simulink model "practica2_3x3sonmem"  (Simulink 7.3)
settings: Solver=ode45  StartTime=0.0  StopTime=10.0  RelTol=1e-3
undefined symbols (not defined in the file or in its folder): p
libraries: simeventsrouting1 x15, simeventssink1 x12, simeventsgenerators1 x6, simeventsqueue1 x6, simeventsattributes2 x6, simeventstiming1 x6, simeventsgates1 x3, simeventsserver1 x3
settings Model: Creator=usuario  LastModifiedBy=usuario
settings SimEventsCC: propDiagAttribOutput=1  propDiagFcnCallOutput=1  propDiagStatOutput=0

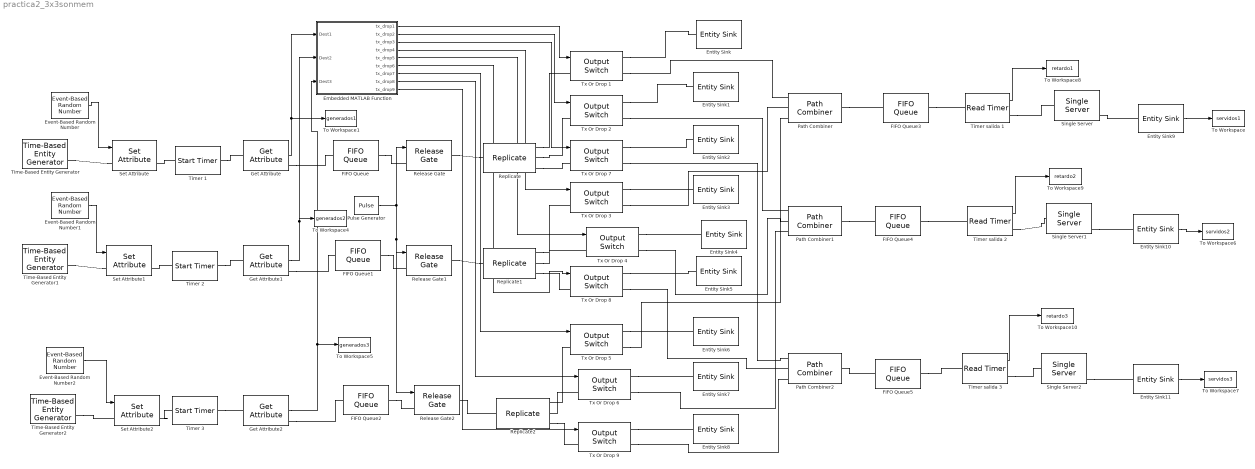
== system practica2_3x3sonmem ==
  Embedded MATLAB Function : Stateflow chart
  Entity Sink{,1..8} (9 alike) : simeventssink1/Entity Sink  Priority=1  SystemSampleTime=-1  AvailableForArrivals=on  StatNumberArrived=Off
  Entity Sink10 : simeventssink1/Entity Sink  Priority=1  SystemSampleTime=-1  AvailableForArrivals=on  StatNumberArrived=On
  Entity Sink11 : simeventssink1/Entity Sink  Priority=1  SystemSampleTime=-1  AvailableForArrivals=on  StatNumberArrived=On
  Entity Sink9 : simeventssink1/Entity Sink  Priority=1  SystemSampleTime=-1  AvailableForArrivals=on  StatNumberArrived=On
  Event-Based Random Number : simeventsgenerators1/Signal Generators/Event-Based Random Number  SystemSampleTime=-1  distribution=Arbitrary discrete  meanExp=1  minUnif=1  maxUnif=1  pOneBern=0.25  pSuccessBino=0.5  numTrialBino=1  meanNorm=0  stdNorm=1  minTri=1  maxTri=3  modeTri=2  thresholdLogn=0  scaleLogn=1  shapeLogn=1  pSuccessGeo=0.5  meanPoiss=1  thresholdLogl=0  scaleLogl=1  thresholdGam=0  scaleGam=1  shapeGam=1  minBeta=0  maxBeta=1  shape1Beta=1  shape2Beta=1  minUnid=0  maxUnid=1  numValueUnid=2  thresholdWbl=0  scaleWbl=1  shapeWbl=1  valueVecCont=[0 1]  cdfVecCont=[0 1]  valueVecDisc=[0 1 2 3]  probVecDisc=[1-p p/3 p/3 p/3]  seed=12345  IsProcessed=on  isConnected=1
  Event-Based Random Number1 : simeventsgenerators1/Signal Generators/Event-Based Random Number  SystemSampleTime=-1  distribution=Arbitrary discrete  meanExp=1  minUnif=1  maxUnif=1  pOneBern=0.25  pSuccessBino=0.5  numTrialBino=1  meanNorm=0  stdNorm=1  minTri=1  maxTri=3  modeTri=2  thresholdLogn=0  scaleLogn=1  shapeLogn=1  pSuccessGeo=0.5  meanPoiss=1  thresholdLogl=0  scaleLogl=1  thresholdGam=0  scaleGam=1  shapeGam=1  minBeta=0  maxBeta=1  shape1Beta=1  shape2Beta=1  minUnid=0  maxUnid=1  numValueUnid=2  thresholdWbl=0  scaleWbl=1  shapeWbl=1  valueVecCont=[0 1]  cdfVecCont=[0 1]  valueVecDisc=[0 1 2 3]  probVecDisc=[1-p p/3 p/3 p/3]  seed=76543  IsProcessed=on  isConnected=1
  Event-Based Random Number2 : simeventsgenerators1/Signal Generators/Event-Based Random Number  SystemSampleTime=-1  distribution=Arbitrary discrete  meanExp=1  minUnif=1  maxUnif=1  pOneBern=0.25  pSuccessBino=0.5  numTrialBino=1  meanNorm=0  stdNorm=1  minTri=1  maxTri=3  modeTri=2  thresholdLogn=0  scaleLogn=1  shapeLogn=1  pSuccessGeo=0.5  meanPoiss=1  thresholdLogl=0  scaleLogl=1  thresholdGam=0  scaleGam=1  shapeGam=1  minBeta=0  maxBeta=1  shape1Beta=1  shape2Beta=1  minUnid=0  maxUnid=1  numValueUnid=2  thresholdWbl=0  scaleWbl=1  shapeWbl=1  valueVecCont=[0 1]  cdfVecCont=[0 1]  valueVecDisc=[0 1 2 3]  probVecDisc=[1-p p/3 p/3 p/3]  seed=89652  IsProcessed=on  isConnected=1
  FIFO Queue : simeventsqueue1/FIFO Queue  Priority=1  SystemSampleTime=-1  Capacity=1  EnableTOPort=off  StatNumberDeparted=Off  StatNumberInBlock=Off  StatPendingEntity=Off  StatAverageWait=Off  StatAverageQueueLength=Off  StatNumberTimedout=Off
  FIFO Queue1 : simeventsqueue1/FIFO Queue  Priority=1  SystemSampleTime=-1  Capacity=1  EnableTOPort=off  StatNumberDeparted=Off  StatNumberInBlock=Off  StatPendingEntity=Off  StatAverageWait=Off  StatAverageQueueLength=Off  StatNumberTimedout=Off
  FIFO Queue2 : simeventsqueue1/FIFO Queue  Priority=1  SystemSampleTime=-1  Capacity=1  EnableTOPort=off  StatNumberDeparted=Off  StatNumberInBlock=Off  StatPendingEntity=Off  StatAverageWait=Off  StatAverageQueueLength=Off  StatNumberTimedout=Off
  FIFO Queue3 : simeventsqueue1/FIFO Queue  Priority=1  SystemSampleTime=-1  Capacity=100  EnableTOPort=off  StatNumberDeparted=Off  StatNumberInBlock=Off  StatPendingEntity=Off  StatAverageWait=Off  StatAverageQueueLength=Off  StatNumberTimedout=Off
  FIFO Queue4 : simeventsqueue1/FIFO Queue  Priority=1  SystemSampleTime=-1  Capacity=100  EnableTOPort=off  StatNumberDeparted=Off  StatNumberInBlock=Off  StatPendingEntity=Off  StatAverageWait=Off  StatAverageQueueLength=Off  StatNumberTimedout=Off
  FIFO Queue5 : simeventsqueue1/FIFO Queue  Priority=1  SystemSampleTime=-1  Capacity=100  EnableTOPort=off  StatNumberDeparted=Off  StatNumberInBlock=Off  StatPendingEntity=Off  StatAverageWait=Off  StatAverageQueueLength=Off  StatNumberTimedout=Off
  Get Attribute : simeventsattributes2/Get Attribute  Priority=1  DialogController=des_ddg_create  DialogControllerArgs=DataTag19  SystemSampleTime=-1  AttributeName=Attribute1  AttributeMissing=Error  AttributeDefaultValue=1  AttributeSendTiming=After entity departure  AttributeTreatAsVector=1  StatNumberDeparted=On  EvaluatedDefaultAttributeValue={[]}
  Get Attribute1 : simeventsattributes2/Get Attribute  Priority=1  DialogController=des_ddg_create  DialogControllerArgs=DataTag21  SystemSampleTime=-1  AttributeName=Attribute1  AttributeMissing=Error  AttributeDefaultValue=1  AttributeSendTiming=After entity departure  AttributeTreatAsVector=1  StatNumberDeparted=On  EvaluatedDefaultAttributeValue={[]}
  Get Attribute2 : simeventsattributes2/Get Attribute  Priority=1  DialogController=des_ddg_create  DialogControllerArgs=DataTag23  SystemSampleTime=-1  AttributeName=Attribute1  AttributeMissing=Error  AttributeDefaultValue=1  AttributeSendTiming=After entity departure  AttributeTreatAsVector=1  StatNumberDeparted=On  EvaluatedDefaultAttributeValue={[]}
  Path Combiner : simeventsrouting1/Path Combiner  Priority=1  SystemSampleTime=-1  NumberInputPorts=3  InputPortPrecedence=IN1 port  InitialSeed=45675  SpecifyEventPriority=off  PriorityPathCombinerPortPrecedenceSelection=4100  StatNumberDeparted=Off  StatLastArrivalPort=Off  EvaluatedNumPorts=3
  Path Combiner1 : simeventsrouting1/Path Combiner  Priority=1  SystemSampleTime=-1  NumberInputPorts=3  InputPortPrecedence=IN1 port  InitialSeed=45675  SpecifyEventPriority=off  PriorityPathCombinerPortPrecedenceSelection=4100  StatNumberDeparted=Off  StatLastArrivalPort=Off  EvaluatedNumPorts=3
  Path Combiner2 : simeventsrouting1/Path Combiner  Priority=1  SystemSampleTime=-1  NumberInputPorts=3  InputPortPrecedence=IN1 port  InitialSeed=45675  SpecifyEventPriority=off  PriorityPathCombinerPortPrecedenceSelection=4100  StatNumberDeparted=Off  StatLastArrivalPort=Off  EvaluatedNumPorts=3
  Pulse Generator : DiscretePulseGenerator  Amplitude=1  Period=10  PulseWidth=5  PhaseDelay=3  SampleTime=0.1
  Release Gate : simeventsgates1/Release Gate  Priority=1  SystemSampleTime=-1  OpenGateUpon=Change in signal from port vc  SignalEdgeOption=Rising  SpecifyEventPriority=off  PriorityGateRelease=2200  StatNumberDeparted=Off
  Release Gate1 : simeventsgates1/Release Gate  Priority=1  SystemSampleTime=-1  OpenGateUpon=Change in signal from port vc  SignalEdgeOption=Rising  SpecifyEventPriority=off  PriorityGateRelease=2200  StatNumberDeparted=Off
  Release Gate2 : simeventsgates1/Release Gate  Priority=1  SystemSampleTime=-1  OpenGateUpon=Change in signal from port vc  SignalEdgeOption=Rising  SpecifyEventPriority=off  PriorityGateRelease=2200  StatNumberDeparted=Off
  Replicate : simeventsrouting1/Replicate  Priority=1  SystemSampleTime=-1  NumberOutputPorts=3  ReplicateEntityWhen=All entity output ports are not blocked  OutputPortPrecedence=OUT1 port  InitialSeed=56789  ActionUponBlocking=Discard entity  StatNumberArrived=Off  StatNumberDeparted=Off  EvaluatedNumPorts=3
  Replicate1 : simeventsrouting1/Replicate  Priority=1  SystemSampleTime=-1  NumberOutputPorts=3  ReplicateEntityWhen=All entity output ports are not blocked  OutputPortPrecedence=OUT1 port  InitialSeed=56789  ActionUponBlocking=Discard entity  StatNumberArrived=Off  StatNumberDeparted=Off  EvaluatedNumPorts=3
  Replicate2 : simeventsrouting1/Replicate  Priority=1  SystemSampleTime=-1  NumberOutputPorts=3  ReplicateEntityWhen=All entity output ports are not blocked  OutputPortPrecedence=OUT1 port  InitialSeed=56789  ActionUponBlocking=Discard entity  StatNumberArrived=Off  StatNumberDeparted=Off  EvaluatedNumPorts=3
  Set Attribute : simeventsattributes2/Set Attribute  Priority=1  DialogController=des_ddg_create  DialogControllerArgs=DataTag34  SystemSampleTime=-1  AttributeFrom=Signal port  AttributeName=Attribute1  AttributeTreatAsVector=1  AttributeValue=1  AttributeCreate=on  StatNumberDeparted=On  EvaluatedAttributeValue={[]}
  Set Attribute1 : simeventsattributes2/Set Attribute  Priority=1  DialogController=des_ddg_create  DialogControllerArgs=DataTag36  SystemSampleTime=-1  AttributeFrom=Signal port  AttributeName=Attribute1  AttributeTreatAsVector=1  AttributeValue=1  AttributeCreate=on  StatNumberDeparted=On  EvaluatedAttributeValue={[]}
  Set Attribute2 : simeventsattributes2/Set Attribute  Priority=1  DialogController=des_ddg_create  DialogControllerArgs=DataTag38  SystemSampleTime=-1  AttributeFrom=Signal port  AttributeName=Attribute1  AttributeTreatAsVector=1  AttributeValue=1  AttributeCreate=on  StatNumberDeparted=On  EvaluatedAttributeValue={[]}
  Single Server : simeventsserver1/Single Server  Priority=1  SystemSampleTime=-1  ServiceTimeFrom=Dialog  ServiceTime=0.99999  AttributeName=ServiceTime  PriorityServiceCompletion=500  PermitPreemption=off  SortingAttributeName=PriorityAttributeName  SortingDirection=Ascending  WriteToAttribute=off  ResidualAttributeName=ResidualServiceTime  CreateAttribute=on  EnableTOPort=off  StatNumberDeparted=On  StatNumberInBlock=Off  StatNumberPreempted=Off  StatPendingEntity=Off  StatAverageWait=Off  StatUtilization=On  StatNumberTimedout=Off
  Single Server1 : simeventsserver1/Single Server  Priority=1  SystemSampleTime=-1  ServiceTimeFrom=Dialog  ServiceTime=0.99999  AttributeName=ServiceTime  PriorityServiceCompletion=500  PermitPreemption=off  SortingAttributeName=PriorityAttributeName  SortingDirection=Ascending  WriteToAttribute=off  ResidualAttributeName=ResidualServiceTime  CreateAttribute=on  EnableTOPort=off  StatNumberDeparted=On  StatNumberInBlock=Off  StatNumberPreempted=Off  StatPendingEntity=Off  StatAverageWait=Off  StatUtilization=On  StatNumberTimedout=Off
  Single Server2 : simeventsserver1/Single Server  Priority=1  SystemSampleTime=-1  ServiceTimeFrom=Dialog  ServiceTime=0.99999  AttributeName=ServiceTime  PriorityServiceCompletion=500  PermitPreemption=off  SortingAttributeName=PriorityAttributeName  SortingDirection=Ascending  WriteToAttribute=off  ResidualAttributeName=ResidualServiceTime  CreateAttribute=on  EnableTOPort=off  StatNumberDeparted=On  StatNumberInBlock=Off  StatNumberPreempted=Off  StatPendingEntity=Off  StatAverageWait=Off  StatUtilization=On  StatNumberTimedout=Off
  Time-Based Entity Generator : simeventsgenerators1/Entity Generators/Time-Based Entity Generator  Priority=1  DialogController=des_ddg_create  DialogControllerArgs=DataTag43  SystemSampleTime=-1  GenerateEntitiesUpon=Intergeneration time from dialog  Distribution=Constant  Minimum=0  Maximum=1  Mean=1  InitialSeed=12345  Period=1  PriorityEntityGeneration=300  GenerateEntityAtSimulationStart=on  ResponseWhenBlocked=Pause generation  ResponseWhenUnblocked=Immediate restart  EntityType=Blank  StatNumberDeparted=On  StatPendingEntity=Off  StatAverageIntergenerationTime=Off
  Time-Based Entity Generator1 : simeventsgenerators1/Entity Generators/Time-Based Entity Generator  Priority=1  DialogController=des_ddg_create  DialogControllerArgs=DataTag45  SystemSampleTime=-1  GenerateEntitiesUpon=Intergeneration time from dialog  Distribution=Constant  Minimum=0  Maximum=1  Mean=1  InitialSeed=12345  Period=1  PriorityEntityGeneration=300  GenerateEntityAtSimulationStart=on  ResponseWhenBlocked=Pause generation  ResponseWhenUnblocked=Immediate restart  EntityType=Blank  StatNumberDeparted=On  StatPendingEntity=Off  StatAverageIntergenerationTime=Off
  Time-Based Entity Generator2 : simeventsgenerators1/Entity Generators/Time-Based Entity Generator  Priority=1  DialogController=des_ddg_create  DialogControllerArgs=DataTag47  SystemSampleTime=-1  GenerateEntitiesUpon=Intergeneration time from dialog  Distribution=Constant  Minimum=0  Maximum=1  Mean=1  InitialSeed=12345  Period=1  PriorityEntityGeneration=300  GenerateEntityAtSimulationStart=on  ResponseWhenBlocked=Pause generation  ResponseWhenUnblocked=Immediate restart  EntityType=Blank  StatNumberDeparted=On  StatPendingEntity=Off  StatAverageIntergenerationTime=Off
  Timer 1 : simeventstiming1/Start Timer  Priority=0  SystemSampleTime=-1  TimerTag=T1  TimerStartedOption=Warn and continue  StatNumberDeparted=Off
  Timer 2 : simeventstiming1/Start Timer  Priority=0  SystemSampleTime=-1  TimerTag=T1  TimerStartedOption=Warn and continue  StatNumberDeparted=Off
  Timer 3 : simeventstiming1/Start Timer  Priority=0  SystemSampleTime=-1  TimerTag=T1  TimerStartedOption=Warn and continue  StatNumberDeparted=Off
  Timer salida 1 : simeventstiming1/Read Timer  Priority=0  SystemSampleTime=-1  TimerTag=T1  TimerModeOption=Error  TimerStop=off  StatNumberDeparted=Off  StatTimerNumberDeparted=Off  StatTimeElapsed=On  StatAverageTimeElapsed=Off
  Timer salida 2 : simeventstiming1/Read Timer  Priority=0  SystemSampleTime=-1  TimerTag=T1  TimerModeOption=Error  TimerStop=off  StatNumberDeparted=Off  StatTimerNumberDeparted=Off  StatTimeElapsed=On  StatAverageTimeElapsed=Off
  Timer salida 3 : simeventstiming1/Read Timer  Priority=0  SystemSampleTime=-1  TimerTag=T1  TimerModeOption=Error  TimerStop=off  StatNumberDeparted=Off  StatTimerNumberDeparted=Off  StatTimeElapsed=On  StatAverageTimeElapsed=Off
  To Workspace : ToWorkspace  VariableName=servidos1  SampleTime=-1  SaveFormat=Array
  To Workspace1 : ToWorkspace  VariableName=generados1  SampleTime=1  SaveFormat=Array
  To Workspace10 : ToWorkspace  VariableName=retardo3  SampleTime=-1  SaveFormat=Array
  To Workspace4 : ToWorkspace  VariableName=generados2  SampleTime=1  SaveFormat=Array
  To Workspace5 : ToWorkspace  VariableName=generados3  SampleTime=1  SaveFormat=Array
  To Workspace6 : ToWorkspace  VariableName=servidos2  SampleTime=-1  SaveFormat=Array
  To Workspace7 : ToWorkspace  VariableName=servidos3  SampleTime=-1  SaveFormat=Array
  To Workspace8 : ToWorkspace  VariableName=retardo1  SampleTime=-1  SaveFormat=Array
  To Workspace9 : ToWorkspace  VariableName=retardo2  SampleTime=-1  SaveFormat=Array
  Tx Or Drop {1..9} (9 alike) : simeventsrouting1/Output Switch  Priority=1  SystemSampleTime=-1  NumberOutputPorts=2  SwitchingCriterion=From signal port p  InitialSeed=34567  AttributeName=Attribute1  InitialConditionsOpt=off  InitialConditions=1  EntityBufferOpt=off  SpecifyEventPriority=off  PriorityOutputSwitchSelectPort=4100  TimeoutPortOpt=off  StatNumberDeparted=Off  StatNumberTimedOut=Off  StatPendingEntity=Off  StatLastDeparturePort=Off  EvaluatedNumPorts=2
  wires:
  Event-Based Random Number/1 -> Set Attribute/1
  Event-Based Random Number1/1 -> Set Attribute1/1
  Pulse Generator/1 -> Release Gate/1, Release Gate1/1, Release Gate2/1
  Event-Based Random Number2/1 -> Set Attribute2/1
  Get Attribute/2 -> Embedded MATLAB Function/1(Dest1), To Workspace1/1
  Get Attribute1/2 -> Embedded MATLAB Function/2(Dest2), To Workspace4/1
  Get Attribute2/2 -> Embedded MATLAB Function/3(Dest3), To Workspace5/1
  Embedded MATLAB Function/1(tx_drop1) -> Tx Or Drop 1/1
  Embedded MATLAB Function/2(tx_drop2) -> Tx Or Drop 2/1
  Embedded MATLAB Function/3(tx_drop3) -> Tx Or Drop 7/1
  Embedded MATLAB Function/4(tx_drop4) -> Tx Or Drop 3/1
  Embedded MATLAB Function/5(tx_drop5) -> Tx Or Drop 4/1
  Embedded MATLAB Function/6(tx_drop6) -> Tx Or Drop 8/1
  Embedded MATLAB Function/7(tx_drop7) -> Tx Or Drop 5/1
  Embedded MATLAB Function/8(tx_drop8) -> Tx Or Drop 6/1
  Embedded MATLAB Function/9(tx_drop9) -> Tx Or Drop 9/1
  Entity Sink9/1 -> To Workspace/1
  Entity Sink10/1 -> To Workspace6/1
  Entity Sink11/1 -> To Workspace7/1
  Timer salida 1/1 -> To Workspace8/1
  Timer salida 2/1 -> To Workspace9/1
  Timer salida 3/1 -> To Workspace10/1
  connections:
  Replicate/RConn1 -- Tx Or Drop 1/LConn1
  FIFO Queue2/RConn1 -- Release Gate2/LConn1
  Replicate1/RConn3 -- Tx Or Drop 8/LConn1
  Replicate1/RConn1 -- Tx Or Drop 3/LConn1
  Timer 2/RConn1 -- Get Attribute1/LConn1
  Replicate/RConn2 -- Tx Or Drop 2/LConn1
  Replicate2/RConn3 -- Tx Or Drop 9/LConn1
  Single Server2/RConn1 -- Entity Sink11/LConn1
  Set Attribute1/RConn1 -- Timer 2/LConn1
  Timer 3/RConn1 -- Get Attribute2/LConn1
  Tx Or Drop 9/RConn1 -- Entity Sink8/LConn1
  Single Server1/RConn1 -- Entity Sink10/LConn1
  Set Attribute2/RConn1 -- Timer 3/LConn1
  Tx Or Drop 8/RConn1 -- Entity Sink5/LConn1
  Tx Or Drop 1/RConn1 -- Entity Sink/LConn1
  Replicate2/RConn2 -- Tx Or Drop 6/LConn1
  Tx Or Drop 7/RConn1 -- Entity Sink2/LConn1
  Timer 1/RConn1 -- Get Attribute/LConn1
  Timer salida 3/RConn1 -- Single Server2/LConn1
  Replicate2/RConn1 -- Tx Or Drop 5/LConn1
  Tx Or Drop 6/RConn1 -- Entity Sink7/LConn1
  Tx Or Drop 3/RConn1 -- Entity Sink3/LConn1
  Timer salida 1/RConn1 -- Single Server/LConn1
  Release Gate2/RConn1 -- Replicate2/LConn1
  Get Attribute/RConn1 -- FIFO Queue/LConn1
  Time-Based Entity Generator/RConn1 -- Set Attribute/LConn1
  Get Attribute2/RConn1 -- FIFO Queue2/LConn1
  Replicate/RConn3 -- Tx Or Drop 7/LConn1
  Single Server/RConn1 -- Entity Sink9/LConn1
  Timer salida 2/RConn1 -- Single Server1/LConn1
  Tx Or Drop 2/RConn1 -- Entity Sink1/LConn1
  Replicate1/RConn2 -- Tx Or Drop 4/LConn1
  Tx Or Drop 4/RConn1 -- Entity Sink4/LConn1
  Tx Or Drop 5/RConn1 -- Entity Sink6/LConn1
  Get Attribute1/RConn1 -- FIFO Queue1/LConn1
  FIFO Queue1/RConn1 -- Release Gate1/LConn1
  Release Gate1/RConn1 -- Replicate1/LConn1
  Release Gate/RConn1 -- Replicate/LConn1
  Time-Based Entity Generator1/RConn1 -- Set Attribute1/LConn1
  FIFO Queue/RConn1 -- Release Gate/LConn1
  Set Attribute/RConn1 -- Timer 1/LConn1
  Time-Based Entity Generator2/RConn1 -- Set Attribute2/LConn1
  Path Combiner/RConn1 -- FIFO Queue3/LConn1
  FIFO Queue3/RConn1 -- Timer salida 1/LConn1
  Path Combiner1/RConn1 -- FIFO Queue4/LConn1
  FIFO Queue4/RConn1 -- Timer salida 2/LConn1
  Path Combiner2/RConn1 -- FIFO Queue5/LConn1
  FIFO Queue5/RConn1 -- Timer salida 3/LConn1
  Tx Or Drop 1/RConn2 -- Path Combiner/LConn1
  Tx Or Drop 2/RConn2 -- Path Combiner1/LConn1
  Tx Or Drop 3/RConn2 -- Path Combiner/LConn2
  Tx Or Drop 5/RConn2 -- Path Combiner/LConn3
  Tx Or Drop 9/RConn2 -- Path Combiner2/LConn3
  Tx Or Drop 7/RConn2 -- Path Combiner2/LConn1
  Tx Or Drop 6/RConn2 -- Path Combiner1/LConn3
  Tx Or Drop 4/RConn2 -- Path Combiner1/LConn2
  Tx Or Drop 8/RConn2 -- Path Combiner2/LConn2

== matlab function Embedded MATLAB Function ==
  data: Dest1 input double; Dest2 input double; tx_drop1 output double; tx_drop2 output double; tx_drop3 output double; tx_drop4 output double; Dest3 input double; tx_drop5 output double; tx_drop6 output double; tx_drop7 output double; tx_drop8 output double; tx_drop9 output double
function [tx_drop1, tx_drop2, tx_drop3, tx_drop4, tx_drop5, tx_drop6, tx_drop7, tx_drop8, tx_drop9] = port_selection_line1(Dest1, Dest2, Dest3)

MatrizPuntosCruce = ones(3,3);

% Se cierran los puntos de cruce en la Matriz de Barras Cruzadas

if (Dest1 ~= 0)                     %Si la celda en la línea 1 no está vacía
    MatrizPuntosCruce(1,Dest1) = 2; % Se cierra el punto de cruce en
                                    % la primera fila
end

if (Dest2 ~= 0)                    %Si la celda en la línea 2 no está vacía
    MatrizPuntosCruce(2,Dest2) = 2;% Se cierra el punto de cruce en
                                   % la segunda fila
end

if (Dest3 ~= 0)                    %Si la celda en la línea 3 no está vacía
    MatrizPuntosCruce(3,Dest3) = 2;% Se cierra el punto de cruce en
                                   % la tercera fila
end


tx_drop1 = MatrizPuntosCruce(1,1);
tx_drop2 = MatrizPuntosCruce(1,2);
tx_drop3 = MatrizPuntosCruce(1,3);
tx_drop4 = MatrizPuntosCruce(2,1);
tx_drop5 = MatrizPuntosCruce(2,2);
tx_drop6 = MatrizPuntosCruce(2,3);
tx_drop7 = MatrizPuntosCruce(3,1);
tx_drop8 = MatrizPuntosCruce(3,2);
tx_drop9 = MatrizPuntosCruce(3,3);
